simulink library "lib_Clutchless_HSC"  (R2017b)
settings: Solver=VariableStepAuto  StartTime=0.0  StopTime=10.0  RelTol=1e-3
undefined symbols (not defined in the file): cal, eng, Engine, ENGTRQ_MSMCH_Degraded_CP, ENGTRQ_MSMCH_ErrCritical_CP, ENGTRQ_MSMCH_LimpHome_CP, gb, mot, tloop
libraries: simulink x83, EC2_libraries x4, powerlib_meascontrol x2, lib_SystemDiag x1, dspsigops x1
(part 6 of 6)

== stateflow chart lib_Clutchless_HSC/Clutchless_HSC/HSC/Powertrain Manager/Torque Distribution/Supervisory  Control  Logic ==
  note: 
  note: Tranmission Shift Level Position (ShftLvrPos):
  state VehOffOrAcc
    en:
    mode=0;
    EnablePrplsn = 0;
    HV_Req=0;
    closeMaincReq=0;
  state VehOn
    en:
    mode = 6;
    HV_Req=1;
  state Close_Contactors
    en:
    closeMaincReq=1;
  state ChgTrans
    en:
    mode=10;
  note: System Power Mode (KeyPos):
  state VehShutdown
    en:
    powerMode = 1;
    EnablePrplsn = 0;
    EngOnReq = 0;
    EngAppReq = 0;
    EnableInverter=0;
    mode=8;
  state Wait
  state Charging
    en:
    mode = 9;
    HV_Req=1;
    closeMaincReq = 1;
    EnablePrplsn = 0;
    EnableInverter = 0;
  state EnablePropulsion
    en:
    mode=7;
    EnablePrplsn = 1;
    EngOnReq=1;
  state HV_Shutdown
    en:
    HV_Req=0;
    closeMaincReq=0;
  state IMG_Shutdown
    en:
    MotTrqReq = 0;
  state VehReady
    en:
    powerMode = 2;
    state EnableMotor
      EnableInverter=1;
    state Eng_Charging_Stat
      en:
      EngOnReq = 1;
      mode=5;
      du:
      MotTrqReq = MotTrqCalc(ShftLvrPos,DrvIntdAxleTrq,EngTrq);
      EngTrq = EngTrqCalc(EngSpd,ShftLvrPos,DrvIntdAxleTrq,TransRatio);
      EngAppReq=drvAPP;
      state Trq = EngTrqCalc(EngSpeed,ShftLvrPos,DrvIntdAxleTrq,TransRatio) [function]
      state MotTrq = MotTrqCalc(ShftLvrPos,DrvIntdAxleTrq,Trq) [function]
      state APP = EngTrq2EngApp(Trq,TransRatio) [function]
    state CD_Mode
      en:
      mode=1;
      state Drive_mode
        en:
        Brkmode=0;
        du:
        MotTrqReq = MotTrqCalc2(drvAPP,ShftLvrPos,DrvIntdAxleTrq,TransRatio,EngTrq);
        EngTrq=EngTrqCalc(EngSpd,drvAPP,VehicleSpeed,ShftLvrPos,DrvIntdAxleTrq,TransRatio);
        EngAppReq=EngTrq2EngApp(EngTrq,TransRatio);
        state MotTrq = MotTrqCalc2(APP,ShftLvrPos,DrvIntdAxleTrq,TransRatio,Trq) [function]
        state Trq = EngTrqCalc(EngSpeed,APP,VehSpd,ShftLvrPos,DrvIntdAxleTrq,TransRatio) [function]
        state APP = EngTrq2EngApp(Trq,TransRatio) [function]
      state Brake_mode
        en:
        EngAppReq=0;
        state Regen_mode
          en:
          Brkmode=1;
          du:
          MotTrqReq=MotTrqCalc1(BrkPdlPos,VehicleSpeed,...
          ShftLvrPos,MotSpd,TransRatio,IntdAxleTrq);
        state No_regen
          en:
          Brkmode=2;
          du:
          MotTrqReq=MotTrqCalc2(ShftLvrPos,TransRatio);
        state Temp_delay
        state Temp_delay1
        state T = MotTrqCalc1(BPP,VehSpd,ShftLvrPos,MotSpeed,TransRatio,IntdAxleTrq) [function]
        state T = MotTrqCalc2(ShftLvrPos,TransRatio) [function]
        (default) -> VehReady.CD_Mode.Brake_mode.No_regen
        VehReady.CD_Mode.Brake_mode.Regen_mode -> VehReady.CD_Mode.Brake_mode.Temp_delay : [RegenBrkDisable||SoC>=80||ABSAtv||Regen_fault]
        VehReady.CD_Mode.Brake_mode.Temp_delay -> VehReady.CD_Mode.Brake_mode.No_regen : after(0.25,sec)
        VehReady.CD_Mode.Brake_mode.Temp_delay1 -> VehReady.CD_Mode.Brake_mode.Regen_mode : after(0.25,sec)
        VehReady.CD_Mode.Brake_mode.No_regen -> VehReady.CD_Mode.Brake_mode.Temp_delay1 : [RegenBrkDisable == 0&&SoC<80&&ABSAtv==0&&Regen_fault==0]
      state Time_delay
      state Time_delay1
      (default) -> VehReady.CD_Mode.Drive_mode
      VehReady.CD_Mode.Drive_mode -> VehReady.CD_Mode.Time_delay : [BrkPdlPos>0&&IntdAxleTrq<0]
      VehReady.CD_Mode.Time_delay -> VehReady.CD_Mode.Brake_mode : after(0.25,sec)
      VehReady.CD_Mode.Time_delay1 -> VehReady.CD_Mode.Drive_mode : after(0.25,sec)
      VehReady.CD_Mode.Brake_mode -> VehReady.CD_Mode.Time_delay1 : [drvAPP>0&&IntdAxleTrq>=0]
    state Eng_Only_Mode
      en:
      EngOnReq = 1;
      mode=66;
      du:
      MotTrqReq = 0;
      closeMaincReq=0;
      EngTrq = EngTrqCalc(drvAPP,EngSpd,ShftLvrPos,DrvIntdAxleTrq,TransRatio);
      EngAppReq=drvAPP;
      state T = EngTrqCalc(APP,EngSpeed,Shifter,DrvIntdAxleTrq,TransRatio) [function]
      state APP = EngTrq2EngApp(T,TransRatio) [function]
    state Sport_Mode
      en:
      mode=4;
      EngOnReq = 1;
      state Brake_mode
        du:
        EngTrq =0;
        EngAppReq = 0;
        state Regen_mode
          en:
          Brkmode=1;
          du:
          MotTrqReq=MotTrqCalc1(BrkPdlPos,VehicleSpeed,...
          ShftLvrPos,MotSpd,IntdAxleTrq,TransRatio);
        state No_regen
          en:
          Brkmode=2;
          du:
          MotTrqReq=0;
        state Temp_delay
        state Temp_delay1
        state T = MotTrqCalc1(BPP,VehSpd,ShftLvrPos,MotSpeed,IntdAxleTrq,TransRatio) [function]
        (default) -> VehReady.Sport_Mode.Brake_mode.No_regen
        VehReady.Sport_Mode.Brake_mode.Regen_mode -> VehReady.Sport_Mode.Brake_mode.Temp_delay : [RegenBrkDisable...
            | ||SoC>=80||ABSAtv||Regen_fault]
        VehReady.Sport_Mode.Brake_mode.Temp_delay -> VehReady.Sport_Mode.Brake_mode.No_regen : after(0.5,sec)
        VehReady.Sport_Mode.Brake_mode.Temp_delay1 -> VehReady.Sport_Mode.Brake_mode.Regen_mode : after(1,sec)
        VehReady.Sport_Mode.Brake_mode.No_regen -> VehReady.Sport_Mode.Brake_mode.Temp_delay1 : [!RegenBrkDisable&&SoC<80&&...
            | ABSAtv==0&&!Regen_fault]
      state Drive_mode
        du:
        MotTrqReq = MotTrqCalc(drvAPP,ShftLvrPos,MotSpd,DrvIntdAxleTrq,TransRatio);
        EngTrq = EngTrqCalc(drvAPP,EngSpd,ShftLvrPos,DrvIntdAxleTrq,TransRatio);
        EngAppReq = EngTrq2EngApp(EngTrq,TransRatio);
      state Time_delay
      state Time_delay1
      state T = MotTrqCalc(APP,Shifter,MotSpeed,DrvIntdAxleTrq,TransRatio) [function]
      state T = EngTrqCalc(APP,EngSpeed,Shifter,DrvIntdAxleTrq,TransRatio) [function]
      state APP = EngTrq2EngApp(Trq,TransRatio) [function]
      (default) -> VehReady.Sport_Mode.Drive_mode
      VehReady.Sport_Mode.Drive_mode -> VehReady.Sport_Mode.Time_delay : [BrkPdlPos>0&&IntdAxleTrq<0]
      VehReady.Sport_Mode.Time_delay -> VehReady.Sport_Mode.Brake_mode
      VehReady.Sport_Mode.Time_delay1 -> VehReady.Sport_Mode.Drive_mode
      VehReady.Sport_Mode.Brake_mode -> VehReady.Sport_Mode.Time_delay1 : [drvAPP>0&&IntdAxleTrq>=0]
    state CS_Mode
      state Engine_Charge
        en:
        mode=2;
        state Drive_Mode
          en:
          Brkmode=0;
          du:
          EngTrq = EngTrqCalc(EngSpd,drvAPP,VehicleSpeed,ShftLvrPos,DrvIntdAxleTrq,TransRatio,SoC);
          EngAppReq = EngTrq2EngApp(EngTrq,TransRatio);
          MotTrqReq = MotTrqCalc2(drvAPP,ShftLvrPos,DrvIntdAxleTrq,TransRatio,SoC,SW_CS_ON,Faked_SoC,EngTrq,MotSpd);
          state APP = EngTrq2EngApp(Trq,TransRatio) [function]
          state [Trq,EngActTRq] = EngTrqCalc(EngSpeed,APP,VehSpd,ShftLvrPos,DrvIntdAxleTrq,TransRatio,SOC) [function]
          state MotTrq = MotTrqCalc2(APP,ShftLvrPos,DrvIntdAxleTrq,TransRatio,SoC,CS_On,Faked_SoC,EngActTrq,MotSpd) [function]
        state Brake_mode1
          en:
          EngAppReq=0.51;
          state No_regen
            en:
            Brkmode=2;
            du:
            MotTrqReq=MotTrqCalc2(ShftLvrPos,TransRatio);
          state Regen_mode
            en:
            Brkmode=1;
            du:
            MotTrqReq=MotTrqCalc1(BrkPdlPos,VehicleSpeed,...
            ShftLvrPos,MotSpd,TransRatio,IntdAxleTrq);
          state Temp_delay
          state Temp_delay1
          state T = MotTrqCalc1(BPP,VehSpd,ShftLvrPos,MotSpeed,TransRatio,IntdAxleTrq) [function]
          state T = MotTrqCalc2(ShftLvrPos,TransRatio) [function]
          (default) -> VehReady.CS_Mode.Engine_Charge.Brake_mode1.No_regen
          VehReady.CS_Mode.Engine_Charge.Brake_mode1.Regen_mode -> VehReady.CS_Mode.Engine_Charge.Brake_mode1.Temp_delay : [RegenBrkDisable||SoC>=80||ABSAtv||Regen_fault]
          VehReady.CS_Mode.Engine_Charge.Brake_mode1.Temp_delay -> VehReady.CS_Mode.Engine_Charge.Brake_mode1.No_regen : after(0.25,sec)
          VehReady.CS_Mode.Engine_Charge.Brake_mode1.Temp_delay1 -> VehReady.CS_Mode.Engine_Charge.Brake_mode1.Regen_mode : after(0.25,sec)
          VehReady.CS_Mode.Engine_Charge.Brake_mode1.No_regen -> VehReady.CS_Mode.Engine_Charge.Brake_mode1.Temp_delay1 : [RegenBrkDisable == 0&&EngSpd>1000&&SoC<80&&ABSAtv==0&&Regen_fault==0]
        state Time_delay3
        state Time_delay2
        (default) -> Drive_Mode
        Drive_Mode -> Time_delay3 : [BrkPdlPos>0 && IntdAxleTrq<0]
        Time_delay3 -> Brake_mode1 : after(0.25,sec)
        Time_delay2 -> Drive_Mode : after(0.25,sec)
        Brake_mode1 -> Time_delay2 : [drvAPP>0&&IntdAxleTrq>=0]
      (default) -> Engine_Charge
    (default) -> (junction 2118)
    (junction 2118) -> Eng_Only_Mode [order 2] : [eSystemStatus==0]
    (junction 2118) -> EnableMotor [order 1] : [eSystemStatus>1&&iceSystemStatus>1]
    EnableMotor -> (junction 1935)
    (junction 1935) -> Eng_Charging_Stat [order 2] : [SW_Engine_ON&&...
        | HoodStatus==0&&ShftLvrPos==1]
    (junction 1935) -> CD_Mode [order 1] : [InverterEnabled==8&&!SW_Engine_ON]
    CD_Mode -> Eng_Only_Mode [order 3] : [(SoC < 0.1 && ...
        | iceSystemStatus == 2)||...
        | (iceSystemStatus==2&&eSystemStatus == 0)]
    CD_Mode -> Sport_Mode [order 1] : [SportModeEnabled == 1&&...
        | iceSystemStatus>1&&eSystemStatus>1]
    Eng_Only_Mode -> CD_Mode [order 2] : [(SoC > CD_SOC_MIN && ...
        | eSystemStatus == 2) || ...
        | (iceSystemStatus == 0&&eSystemStatus)]
    Sport_Mode -> CD_Mode [order 1] : [SportModeEnabled == 0&&iceSystemStatus&&eSystemStatus]
    Sport_Mode -> CS_Mode [order 2] : [SportModeEnabled == 0&&...
        | iceSystemStatus&&eSystemStatus]
    CS_Mode -> Sport_Mode [order 1] : [SportModeEnabled == 1&&...
        | iceSystemStatus&&eSystemStatus]
    Eng_Only_Mode -> CS_Mode [order 1] : [SoC<CS_SOC_MIN&&SoC>0.1&&eSystemStatus>0]
    CS_Mode -> Eng_Only_Mode [order 2] : [SoC < 0.1||...
        | (iceSystemStatus==2&&eSystemStatus==0)]
    CD_Mode -> CS_Mode [order 2] : [(SW_CS_ON&&iceSystemStatus && ...
        | eSystemStatus)||...
        | SoC <CS_SOC_MIN&&iceSystemStatus == 2 && ...
        | eSystemStatus == 2]
    CS_Mode -> CD_Mode [order 3] : [(!SW_CS_ON&&SoC > CD_SOC_MIN&&...
        | eSystemStatus == 2) || ...
        | iceSystemStatus == 0]
  VehOffOrAcc -> EnablePropulsion [order 2] : [KeyPos==3&&BrkPdlPos>10&&ShftLvrPos==1&&(~eSystemStatus&&iceSystemStatus)]
  VehOffOrAcc -> VehOn [order 1] : [KeyPos>= 1&&(eSystemStatus||iceSystemStatus)]
  (default) -> VehOffOrAcc
  VehOn -> VehOffOrAcc [order 2] : [KeyPos<1]
  VehOn -> Close_Contactors [order 1] : [InverterEnabled==3]
  Close_Contactors -> VehOffOrAcc [order 3] : [KeyPos < 1]
  ChgTrans -> VehOffOrAcc [order 1] : [plugged==0]
  VehOffOrAcc -> ChgTrans [order 3] : [plugged]
      | {HV_Req=1;}
  VehShutdown -> VehOffOrAcc : after(1,sec)...
      | [plugged==0]
  Wait -> VehOffOrAcc [order 1] : after(3,sec)[plugged==0]
  ChgTrans -> Charging [order 2] : after(4,sec)...
      | [INV_State==3]
  Close_Contactors -> Charging [order 2] : [plugged]
  Close_Contactors -> EnablePropulsion [order 1] : [KeyPos==3&&BrkPdlPos>10&&...
      | ShftLvrPos==1]
  Charging -> Wait : [plugged==0]
  Wait -> Charging [order 2] : after(3,sec)[plugged==1]
  HV_Shutdown -> VehShutdown : [InverterEnabled==3]
  EnablePropulsion -> Charging [order 2] : [plugged]
  IMG_Shutdown -> HV_Shutdown : [MotSpd<10&&ShftLvrPos==1]
  EnablePropulsion -> VehReady [order 1] : after(0.5,sec)
  VehReady -> Charging [order 1] : [plugged]
  VehReady -> IMG_Shutdown [order 2] : [KeyPos < 2 ...
      | ||(eSystemStatus==0&&...
      | iceSystemStatus==0)]
  data: Trq function_output; EngSpeed function_input; ShftLvrPos function_input; DrvIntdAxleTrq function_input; TransRatio function_input; MotTrq function_output; ShftLvrPos function_input; DrvIntdAxleTrq function_input; Trq function_input; Trq function_input; APP function_output; TransRatio function_input; APP function_input; MotTrq function_output; ShftLvrPos function_input; DrvIntdAxleTrq function_input; TransRatio function_input; Trq function_input; Trq function_output; EngSpeed function_input; APP function_input; VehSpd function_input; ShftLvrPos function_input; DrvIntdAxleTrq function_input; TransRatio function_input; Trq function_input; APP function_output; TransRatio function_input; T function_output; BPP function_input; VehSpd function_input; ShftLvrPos function_input; MotSpeed function_input; TransRatio function_input; IntdAxleTrq function_input; T function_output; ShftLvrPos function_input; TransRatio function_input; APP function_input; EngSpeed function_input; T function_output; Shifter function_input; DrvIntdAxleTrq function_input; TransRatio function_input; T function_input; APP function_output; TransRatio function_input; T function_output; BPP function_input; VehSpd function_input; ShftLvrPos function_input; MotSpeed function_input; IntdAxleTrq function_input; TransRatio function_input; T function_output; APP function_input; Shifter function_input; MotSpeed function_input; DrvIntdAxleTrq function_input; TransRatio function_input; APP function_input; EngSpeed function_input; T function_output; Shifter function_input; DrvIntdAxleTrq function_input; TransRatio function_input; Trq function_input; APP function_output; TransRatio function_input; temp local double; Trq function_input; APP function_output; TransRatio function_input; Trq function_output; EngSpeed function_input; APP function_input; VehSpd function_input; ShftLvrPos function_input; DrvIntdAxleTrq function_input; TransRatio function_input; SOC function_input; EngActTRq function_output; APP function_input; MotTrq function_output; ShftLvrPos function_input; DrvIntdAxleTrq function_input; TransRatio function_input; SoC function_input; CS_On function_input; Faked_SoC function_input; EngActTrq function_input; MotSpd function_input; T function_output; BPP function_input; VehSpd function_input; ShftLvrPos function_input; MotSpeed function_input; TransRatio function_input; IntdAxleTrq function_input; T function_output; ShftLvrPos function_input; TransRatio function_input; data local double; SportModeEnabled input boolean; TransEstGear input int8; mode output int8; powerMode output int8; closeMaincReq output double; EnablePrplsn output boolean; KeyPos input int8; BrkPdlPos input double; drvAPP input double; VehicleSpeed input double; EngSpd input double; MotSpd input double; ShftLvrPos input int8; EngAppReq output double; EngOnReq output boolean; MotTrqReq output double; EnableInverter output boolean; InverterEnabled input double; plugged input double; CD_SOC_MIN input double; CS_SOC_MIN input double; CS_SOC_MAX input double; EngRunAtv input boolean; SoC input double; EngTrq output double; DrvIntdAxleTrq input double; IntdAxleTrq input double; Faked_SoC input double; TransRatio input double; HV_Req output double; SW_CS_ON input boolean; SW_Engine_ON input boolean; RegenBrkDisable input boolean; Chg output double; Brkmode output double; Drvmode output double; eSystemStatus input; iceSystemStatus input; Drv_Mode local double; ABSAtv input boolean; Regen_fault input boolean; EngFdbkTrq input double; EngCtlTmp input; ClutchEngage output double; INV_State input; HoodStatus input

== stateflow chart lib_Clutchless_HSC/Clutchless_HSC/HSC/Camaro Fault Detection/Component Diagnostic/Transmission Component Diagnostic/TCM_CompDia ==
  state TCM_Offline
    en: TCM_Status=0;
  state TCM_Limited [commented out]
    en: TCM_Status=1;
  state TCM_Online
    en: TCM_Status=2;
  (default) -> TCM_Offline
  TCM_Online -> TCM_Offline : [~TCMRollingAliveActive_SigValid||...
      | ~LvrPosTrnsShft_SigValid||...
      | ~TransEstGear_SigValid||...
      | ~LockupCmd_SigValid||VehDirFault]
  TCM_Offline -> TCM_Online : [TCMRollingAliveActive_SigValid&&...
      | LvrPosTrnsShft_SigValid&&TransEstGear_SigValid&&...
      | LockupCmd_SigValid&&VehDirFault==0]
  TCM_Limited -> TCM_Online [commented out]
  TCM_Online -> TCM_Limited [commented out]
  data: TCM_Status output; TCMRollingAliveActive_SigValid input; LvrPosTrnsShft_SigValid input; TransEstGear_SigValid input; LockupCmd_SigValid input; VehDirFault input

== stateflow chart lib_Clutchless_HSC/Clutchless_HSC/HSC/Camaro Fault Detection/Input Conversions/TCM_Conversions/TCM_RollinAliveCounter/Rolling Alive Counter1 ==
  state RollingAliveCounter
    state Count1
      en: RollingAliveCnt=0;
    state Count2
      en: RollingAliveCnt=1;
    state Count3
      en: RollingAliveCnt=2;
    state Count4
      en: RollingAliveCnt=3;
    (default) -> Count1
    Count4 -> Count1 : after(0.01,sec)
    Count1 -> Count2 : after(0.01,sec)
    Count2 -> Count3 : after(0.01,sec)
    Count3 -> Count4 : after(0.01,sec)
  data: RollingAliveCnt output double

== stateflow chart lib_Clutchless_HSC/Clutchless_HSC/HSC/Camaro Fault Detection/Signal Diagnostic/Engine Signal Diagnostic/Engine_Temp[DegC] ==
  state AboveMax
    en: EngTempRange=3;
  state HighRange
    en: EngTempRange=2;
  state NormalRange
    en: EngTempRange=1;
  HighRange -> AboveMax [order 2] : [Engine_Temp_DegC>120]
  AboveMax -> HighRange : [Engine_Temp_DegC<120]
  NormalRange -> HighRange [order 1] : [Engine_Temp_DegC>100&&Engine_Temp_DegC<120]
  HighRange -> NormalRange [order 1] : [Engine_Temp_DegC<=100]
  NormalRange -> NormalRange [order 2] : [clearFaults==1]
      | {EngTempRange=1;}
  (default) -> NormalRange
  data: clearFaults input; Engine_Temp_DegC input; EngTempRange output; data local

== stateflow chart lib_Clutchless_HSC/Clutchless_HSC/HSC/Powertrain Manager/Thermal Manager/ESS Pump Manger/Chart1 ==
  state ESS_Pump [parallel]
    settings: executionOrder=1
    state pump_state_0
      entry: ESS_pump_control=0;
    state pump_low_State_1
      entry: ESS_pump_control=30;
    state pump_transition_3_to_0
    state pump_transition_2_to_0
    state pump_high_State_3
      entry: ESS_pump_control=90;
    state pump_medi_State_2
      entry: ESS_pump_control=60;
    pump_state_0 -> pump_low_State_1 : [(ESS_temp>=ESS_Temp_State_1_Thrs)&&SysPowMod>0]
    (default) -> pump_state_0
    pump_low_State_1 -> pump_state_0 [order 1] : [(ESS_temp<ESS_Temp_State_1_Thrs&&after(10,sec))||SysPowMod==0 ]
    pump_transition_2_to_0 -> pump_state_0 : after(15,sec)
    pump_transition_3_to_0 -> pump_state_0 : after(30,sec)
    pump_low_State_1 -> pump_medi_State_2 [order 2] : [ESS_temp>=ESS_Temp_State_2_Thrs]
    pump_medi_State_2 -> pump_low_State_1 [order 1] : [ESS_temp<ESS_Temp_State_2_Thrs&&after(10,sec)]
    pump_high_State_3 -> pump_transition_3_to_0 [order 2] : [SysPowMod==0]
    pump_medi_State_2 -> pump_transition_2_to_0 [order 3] : [SysPowMod==0]
    pump_medi_State_2 -> pump_high_State_3 [order 2] : [ESS_temp>=ESS_Temp_State_3_Thrs]
    pump_high_State_3 -> pump_medi_State_2 [order 1] : [ESS_temp<ESS_Temp_State_3_Thrs&&after(10,sec)]
  state ESS_comp [parallel]
    settings: executionOrder=2
    state Comp_off
      entry:
      ESS_comp=0;
      ESS_val=0;
      ESS_comp_Enable = 1;
    state Comp_on
      entry:
      ESS_comp=10;
      ESS_val=1;
      ESS_comp_Enable = 0;
    (default) -> Comp_off
    Comp_off -> Comp_on : [(ESS_CltTemp>=ESS_Comp_TempThrs)&&SysPowMod>0]
    Comp_on -> Comp_off : [(ESS_CltTemp<ESS_Comp_TempThrs&&after(25,sec))&&SysPowMod==0]
  data: ESS_temp input; ESS_comp output; ESS_pump_control output; ESS_val output; ESS_Temp_State_1_Thrs input double =15; ESS_Temp_State_2_Thrs input double; ESS_Temp_State_3_Thrs input double; ESS_Comp_TempThrs input double; ESS_CltTemp input; ESS_comp_Enable output; SysPowMod input

== stateflow chart lib_Clutchless_HSC/Clutchless_HSC/HSC/Powertrain Manager/Thermal Manager/MotInv Pump Manger/MCUPump_Manager ==
  state Pump_Off
    entry: MotInvpump_control=0;
  state Pump_transition_2_to_off
  state Pump_High_State_2
    entry: MotInvpump_control=90;
  state Pump_Low_State_1
    entry: MotInvpump_control=60;
  (default) -> Pump_Off
  Pump_transition_2_to_off -> Pump_Off : after(30,sec)
  Pump_Off -> Pump_Low_State_1 : [(Motor_temp>=Mot_Temp_State_1_Thrs||MCU_temp>=MCU_Temp_State_1_Thrs)&&after(10,sec)&&SysPowMod>0]
  Pump_Low_State_1 -> Pump_Off [order 2] : [((Motor_temp<Mot_Temp_State_1_Thrs)&&(MCU_temp<MCU_Temp_State_1_Thrs)&&after(10,sec))||SysPowMod==0]
  Pump_High_State_2 -> Pump_transition_2_to_off [order 2] : [SysPowMod==0]
  Pump_Low_State_1 -> Pump_High_State_2 [order 1] : [(Motor_temp>=Mot_Temp_State_2_Thrs||MCU_temp>=MCU_Temp_State_2_Thrs)&&after(10,sec)]
  Pump_High_State_2 -> Pump_Low_State_1 [order 1] : [(Motor_temp<Mot_Temp_State_2_Thrs&&MCU_temp<MCU_Temp_State_2_Thrs)&&(after(10,sec))]
  data: MotInvpump_control output; Motor_temp input; MCU_temp input; MCU_Temp_State_1_Thrs input double; Mot_Temp_State_1_Thrs input double; MCU_Temp_State_2_Thrs input double; Mot_Temp_State_2_Thrs input double; SysPowMod input
